simulink model "dab_bidirectional_converter_model"  (R2024a)
settings: Solver=ode23tb  StartTime=0.0  StopTime=0.5  MaxStep=1e-3  RelTol=1e-3  EnableMultiTasking=on
PreLoadFcn:
  | DualActiveBridgeConverterData
undefined symbols (not defined in the file): Ts_Power
libraries: spsMosfetLib x8, spsSeriesRLCBranchLib x7, spsVoltageMeasurementLib x5, spsCurrentMeasurementLib x3, simulink_extras x2, spsSawtoothGeneratorLib x2, spsMeanLib x2, spsDCVoltageSourceLib x2, spsLinearTransformerLib x1, slpidlib x1, spsStairGeneratorLib x1, spspowerguiLib x1
settings Model: SimulationMode=accelerator  Creator=The MathWorks, Inc.  LastModifiedBy=hamza
settings SolverCC: AlgebraicLoopSolver=TrustRegion
settings DataIOCC: LimitDataPoints=on  SaveFormat=Array  SaveOutput=off  DSMLogging=off  SaveTime=off  ReturnWorkspaceOutputs=off
settings OptimizationCC: LifeSpan=inf
settings DebuggingCC: SaveWithParameterizedLinksMsg=none  UnderspecifiedInitializationDetection=Classic  MergeDetectMultiDrivingBlocksExec=none  SolverPrmCheckMsg=warning  FcnCallInpInsideContextMsg=warning  UnconnectedInputMsg=warning  UnconnectedOutputMsg=warning  UnconnectedLineMsg=warning  StateNameClashWarn=warning  SubsystemReferenceDiagnosticForUnitTest=warning  SFUnexpectedBacktrackingDiag=warning  SFNoUnconditionalDefaultTransitionDiag=warning  SFExecutionAtInitializationDiag=none  ArithmeticOperatorsInVariantConditions=warning
settings HardwareCC: ProdBitPerPointer=32  ProdBitPerSizeT=32  ProdBitPerPtrDiffT=32  ProdLargestAtomicFloat=None  ProdIntDivRoundTo=Undefined  ProdEndianess=Unspecified  ProdWordSize=32  ProdHWDeviceType=32-bit Generic  TargetHWDeviceType=32-bit Generic
settings ModelReferenceCC: EnableRefExpFcnMdlSchedulingChecks=on  PropagateSignalLabelsOutOfModel=off
settings SFSimCC: SimUseLocalCustomCode=off  CustomCodeUndefinedFunction=UseInterfaceOnly
settings RTWCC: RTWUseLocalCustomCode=off  GPUComputeCapability=3.5  DLArmComputeVersion=19.05
settings CodeAppCC: StateflowObjectComments=on
settings GRTTargetCC: TargetFcnLib=ansi_tfl_tmw.mat  TargetLangStandard=C89/C90 (ANSI)  CombineOutputUpdateFcns=off  GRTInterface=on
settings ConfigComp: CovMetricSettings=dw  CovSaveCumulativeToWorkspaceVar=on  CovSaveSingleToWorkspaceVar=on  CovExternalEMLEnable=off  CovSFcnEnable=off

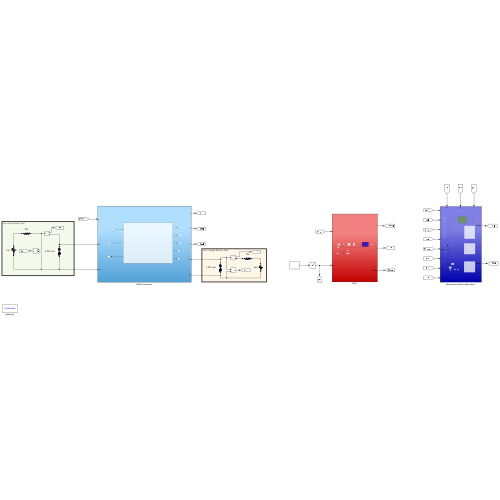
[thumbnail: Simulink's stored preview of the top-level diagram]
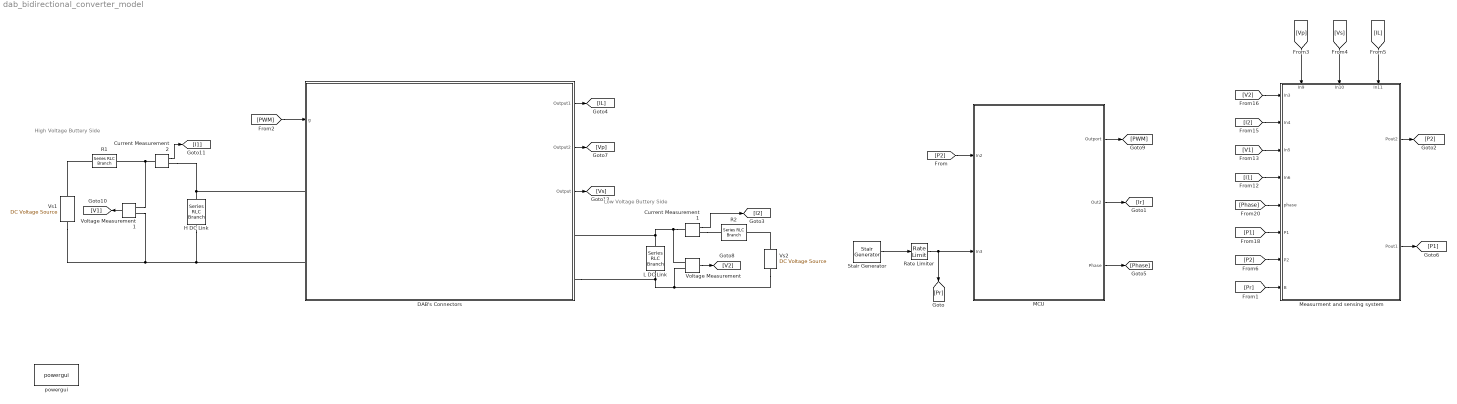
== system dab_bidirectional_converter_model ==
  note: Low Voltage Buttery Side
  note: High Voltage Buttery Side
  Current Measurement1 : spsCurrentMeasurementLib/Current Measurement  PhasorSimulation=off  OutputType=Complex  PSBequivalent=0
  Current Measurement2 : spsCurrentMeasurementLib/Current Measurement  PhasorSimulation=off  OutputType=Complex  PSBequivalent=0
  "DAB's Connectors " : Subsystem
  H DC Link : spsSeriesRLCBranchLib/Series RLC Branch  LConnTagsString=__new0  RConnTagsString=__new0  BranchType=RC  Resistance=1e-3  Inductance=1  SetiL0=off  InitialCurrent=0  Capacitance=100e-5  Setx0=off  InitialVoltage=0  Measurements=None
  L DC Link : spsSeriesRLCBranchLib/Series RLC Branch  LConnTagsString=__new0  RConnTagsString=__new0  BranchType=RC  Resistance=1e-3  Inductance=1  SetiL0=off  InitialCurrent=0  Capacitance=100e-5  Setx0=off  InitialVoltage=0  Measurements=None
  MCU : Subsystem
  Measurment and sensing system : Subsystem
      settings: PortSchema="{\"entries\":[{\"content\":{\"sides\":[{\"content\":{\"connectorIds\":[\"In1\",\"In2\",\"In3\",\"In4\",\"In5\",\"In6\",\"In7\",\"In8\"]},\"type\":\"ConnectorPlacement.EquallySpacedRectSide\",\"uuid\":\"21238e19-9896-4fd6-b727-7e2844941531\"},{\"content\":{\"connectorIds\":[\"Out1\",\"Out2\"],\"side\":\"RIGHT\"},\"type\":\"ConnectorPlacement.EquallySpacedRectSide\",\"uuid\":\"ba89ef00-1c8d-4ed8-ad10-17dc1dc7ec4f\"},{\"content\":{\"connectorIds\":[\"In9\",\"In10\",\"In11\"],\"side\":\"TOP\"},\"type\":\"ConnectorPlacement.EquallySpacedRectSide\",\"uuid\":\"e390a5d7-e81e-44f7-bbae-e4ebff839666\"}]},\"type\":\"ConnectorPlacement.EquallySpacedConnector\",\"uuid\":\"e20906e7-f3d4-4f84-9623-f1df5eb2e679\"}],\"packageUris\":[\"http://schema.mathworks.com/mf0/Connector/R2020b\"],\"version\":\"1.0\"}"
  R1 : spsSeriesRLCBranchLib/Series RLC Branch  LConnTagsString=__new0  RConnTagsString=__new0  BranchType=R  Resistance=20e-3  Inductance=1  SetiL0=off  InitialCurrent=0  Capacitance=1  Setx0=off  InitialVoltage=0  Measurements=None
  R2 : spsSeriesRLCBranchLib/Series RLC Branch  LConnTagsString=__new0  RConnTagsString=__new0  BranchType=R  Resistance=60e-3  Inductance=100e-6  SetiL0=off  InitialCurrent=0  Capacitance=1  Setx0=off  InitialVoltage=0  Measurements=None
  Rate Limiter : RateLimiter  RisingSlewLimit=50  FallingSlewLimit=-50  SampleTimeMode=inherited
  Stair Generator : spsStairGeneratorLib/Stair Generator  t=[0, 0.2]  e=[2 , -2.1]  Ts=0
  Voltage Measurement : spsVoltageMeasurementLib/Voltage Measurement  PhasorSimulation=off  OutputType=Complex  PSBequivalent=0
  Voltage Measurement1 : spsVoltageMeasurementLib/Voltage Measurement  PhasorSimulation=off  OutputType=Complex  PSBequivalent=0
  Vs1 : spsDCVoltageSourceLib/DC Voltage Source  Amplitude=400  Measurements=None
  Vs2 : spsDCVoltageSourceLib/DC Voltage Source  Amplitude=45  Measurements=None
  powergui : spspowerguiLib/powergui  Priority=1  SimulationMode=Continuous  SampleTime=Ts_Power  frequency=60  Iterations=50  frequencyindice=0  Pbase=100e6  ErrMax=1e-4  UnitsV=kV  UnitsW=MW  buscounter=0  FunctionMessages=off  echomessages=off  EnableUseOfTLC=off  CurrentSourceSwitches=on  DisableSnubberDevices=off  DisableRonSwitches=off  DisableVfSwitches=off  DisplayEquations=off  AutomaticDiscreteSolvers=off  SolverType=Tustin/Backward Euler (TBE)  Interpol=off  ExternalGateDelay=off  methode=off  Ts=10  x0status=blocks  SPID=on  SwTol=0  HookPort=off  NonlinearTolerance=1e-4  nMaxIteration=100  ContinueOnMaxIteration=off  RestoreLinks=warning  ResistiveCurrentMeasurement=off  Frange=[0:2:500]  Ylog=off  Xlog=on  ShowGrid=off  save=off  variable=ZData  structure=0  ZoomFFT=off  StartTime=0.0  cycles=1  DisplayStyle=1  fundamental=60  FreqAxis=off  MaxFrequency=1000  frequencyindicesteady=1  RmsSteady=1  display=off
  wires:
  [V2] -> Measurment and sensing system/1(In3)
  [I2] -> Measurment and sensing system/2(In4)
  [V1] -> Measurment and sensing system/3(In5)
  [I1] -> Measurment and sensing system/4(In6)
  [Phase] -> Measurment and sensing system/5(phase)
  [P1] -> Measurment and sensing system/6(P1)
  [P2] -> Measurment and sensing system/7(P2)
  Measurment and sensing system/1(Pout2) -> [P2]
  Measurment and sensing system/2(Pout1) -> [P1]
  [P2] -> MCU/1(In2)
  MCU/1(Outport) -> [PWM]
  MCU/3(Phase) -> [Phase]
  [PWM] -> "DAB's Connectors "/1(g)
  Current Measurement2/1 -> [I1]
  MCU/2(Out2) -> [Ir]
  "DAB's Connectors "/1(Output1) -> [IL]
  "DAB's Connectors "/2(Output2) -> [Vp]
  "DAB's Connectors "/3(Output) -> [Vs]
  [Vs] -> Measurment and sensing system/10(In10)
  [Vp] -> Measurment and sensing system/9(In9)
  [IL] -> Measurment and sensing system/11(In11)
  Stair Generator/1 -> Rate Limiter/1
  Rate Limiter/1 -> MCU/2(In3), [Pr]
  [Pr] -> Measurment and sensing system/8(B)
  Voltage Measurement1/1 -> [V1]
  Current Measurement1/1 -> [I2]
  Voltage Measurement/1 -> [V2]
  connections:
  Current Measurement2/RConn1 -- "DAB's Connectors "/LConn1 -- H DC Link/RConn1
  H DC Link/LConn1 -- Voltage Measurement1/LConn2 -- Vs1/LConn1 -- "DAB's Connectors "/LConn2
  R1/LConn1 -- Voltage Measurement1/LConn1 -- Current Measurement2/LConn1
  R1/RConn1 -- Vs1/RConn1
  Current Measurement1/LConn1 -- L DC Link/RConn1 -- "DAB's Connectors "/RConn1 -- Voltage Measurement/LConn1
  Voltage Measurement/LConn2 -- "DAB's Connectors "/RConn2 -- L DC Link/LConn1 -- Vs2/LConn1
  Vs2/RConn1 -- R2/LConn1
  Current Measurement1/RConn1 -- R2/RConn1

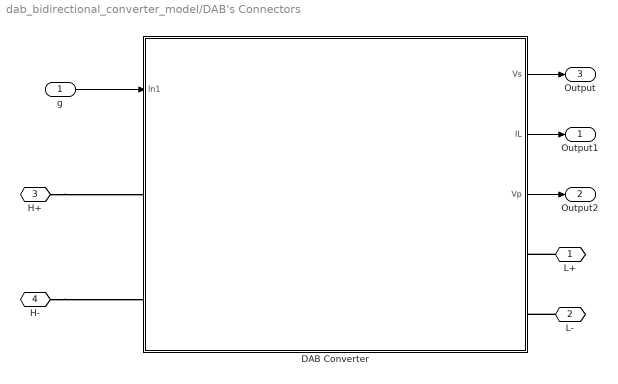
== system dab_bidirectional_converter_model/DAB's Connectors  ==
  g : Inport
  DAB Converter : Subsystem
  L+ : PMIOPort  Side=Right
  L- : PMIOPort  Port=2  Side=Right
  H+ : PMIOPort  Port=3  Side=Left
  H- : PMIOPort  Port=4  Side=Left
  Output1 : Outport
  Output2 : Outport  Port=2
  Output : Outport  Port=3
  wires:
  g/1 -> DAB Converter/1(In1)
  DAB Converter/1(Vs) -> Output/1
  DAB Converter/2(IL) -> Output1/1
  DAB Converter/3(Vp) -> Output2/1
  connections:
  H+/RConn1 -- DAB Converter/LConn1
  H-/RConn1 -- DAB Converter/LConn2
  L-/RConn1 -- DAB Converter/RConn2
  L+/RConn1 -- DAB Converter/RConn1

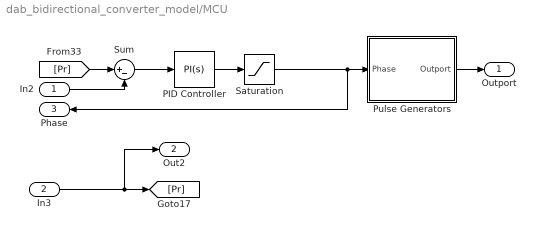
== system dab_bidirectional_converter_model/MCU ==
  In2 : Inport
  In3 : Inport  Port=2
  PID Controller : slpidlib/PID Controller  Controller=PI  Form=Parallel  TimeDomain=Continuous-time  UseExternalTs=off  SampleTime=-1  IntegratorMethod=Forward Euler  FilterMethod=Forward Euler  ControllerParametersSource=internal  P=0.1  I=600  UseKiTs=off  D=0  UseExternalDerivativeSource=off  N=100  UseFilter=on  TunerSelectOption=Transfer Function Based (PID Tuner App)  InitialConditionSource=internal  InitialConditionForIntegrator=0  InitialConditionForFilter=0  DifferentiatorICPrevScaledInput=0  ExternalReset=none  TrackingMode=off  Kt=1  LimitOutput=off  SatLimitsSource=internal  UpperSaturationLimit=inf  LowerSaturationLimit=-inf  LinearizeAsGain=on  AntiWindupMode=none  Kb=1  LimitIntegrator=off  UpperIntegratorSaturationLimit=inf  LowerIntegratorSaturationLimit=-inf  POutMin=[]  POutMax=[]  IOutMin=[]  IOutMax=[]  DOutMin=[]  DOutMax=[]  NOutMin=[]  NOutMax=[]  SumOutMin=[]  SumOutMax=[]  SaturationOutMin=[]  SaturationOutMax=[]  PParamMin=[]  PParamMax=[]  IParamMin=[]  IParamMax=[]  DParamMin=[]  DParamMax=[]  NParamMin=[]  NParamMax=[]  KbParamMin=[]  KbParamMax=[]  KtParamMin=[]  KtParamMax=[]  KbOutMin=[]  KbOutMax=[]  KtOutMin=[]  KtOutMax=[]  IntegratorOutMin=[]  IntegratorOutMax=[]  FilterOutMin=[]  FilterOutMax=[]  SumI1OutMin=[]  SumI1OutMax=[]  SumI2OutMin=[]  SumI2OutMax=[]  SumI3OutMin=[]  SumI3OutMax=[]  SumI4OutMin=[]  SumI4OutMax=[]  SumDOutMin=[]  SumDOutMax=[]  DifferentiatorOutMin=[]  DifferentiatorOutMax=[]  FilterDiffOutCoefMin=[]  FilterDiffOutCoefMax=[]  ReciprocalOutMin=[]  ReciprocalOutMax=[]  SumDenOutMin=[]  SumDenOutMax=[]  SumNumOutMin=[]  SumNumOutMax=[]  DivideOutMin=[]  DivideOutMax=[]  UdiffTsProdOutMin=[]  UdiffTsProdOutMax=[]  NTsProdOutMin=[]  NTsProdOutMax=[]  UintegralTsProdOutMin=[]  UintegralTsProdOutMax=[]  UngainTsProdOutMin=[]  UngainTsProdOutMax=[]  ClampingZeroOutDataTypeStr=Inherit: Inherit via back propagation  ClampingZeroOutMin=[]  ClampingZeroOutMax=[]  FilterDenConstantOutDataTypeStr=Inherit: Inherit via back propagation  FilterDenConstantOutMin=[]  FilterDenConstantOutMax=[]  PCopyOutDataTypeStr=Inherit: Inherit via back propagation  PCopyOutMin=[]  PCopyOutMax=[]  NCopyOutDataTypeStr=Inherit: Inherit via back propagation  NCopyOutMin=[]  NCopyOutMax=[]  IntegratorContinuousStateAttributes=''  IntegratorStateMustResolveToSignalObject=off  IntegratorRTWStateStorageClass=Auto  FilterContinuousStateAttributes=''  FilterStateMustResolveToSignalObject=off  FilterRTWStateStorageClass=Auto  ParallelPVariant=InternalParameters  IdealPVariant=Disabled  IVariant=InternalParameters  DVariant=Disabled  IntegratorVariant=Continuous  SatVariant=Disabled  AWVariant=Passthrough  PCopyVariant=Disabled  TRVariant=Disabled  FdbkBlocksVariant=Forward  IdealPFdbkVariant=Disabled  SatFdbkVariant=Disabled  DerivativeFilterVariant=Disabled  NVariant=Disabled  NCopyVariant=Disabled_SignalSpec  FilterICVariant=Disabled  IntegratorICVariant=InternalICs  ExternalResetVariant=Disabled  TRSumVariant=Passthrough  SumFdbkVariant=Disabled  SumVariant=Sum_PI  TsampFilterVariant=InternalTs  TsampNgainVariant=Passthrough  TsampIntegralVariant=Disabled_SignalSpec  ExternalSaturationOutDataTypeStr=Inherit: Same as second input  DerivativeSourceVariant=Disabled
  Pulse Generators : Subsystem
  Saturation : Saturate  UpperLimit=35  LowerLimit=-35
  Sum : Sum  Inputs=|+-
  Outport : Outport
  Out2 : Outport  Port=2
  Phase : Outport  Port=3
  wires:
  In3/1 -> Out2/1, [Pr]
  Pulse Generators/1(Outport) -> Outport/1
  [Pr] -> Sum/1
  In2/1 -> Sum/2
  PID Controller/1 -> Saturation/1
  Sum/1 -> PID Controller/1
  Saturation/1 -> Phase/1, Pulse Generators/1(Phase)

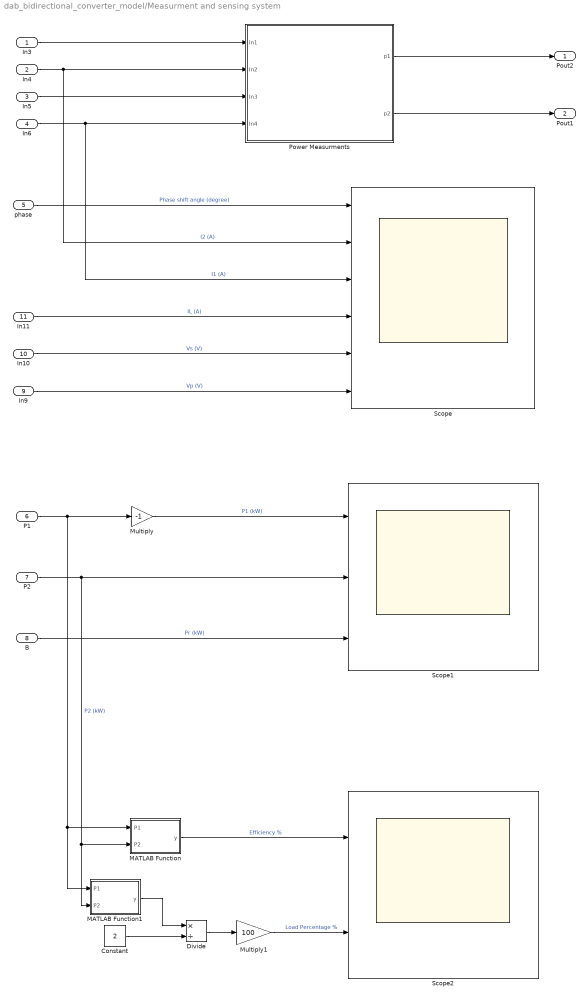
== system dab_bidirectional_converter_model/Measurment and sensing system ==
  In3 : Inport
  In4 : Inport  Port=2
  In5 : Inport  Port=3
  In6 : Inport  Port=4
  phase : Inport  Port=5
  P1 : Inport  Port=6
  P2 : Inport  Port=7
  B : Inport  Port=8
  In9 : Inport  Port=9
  In10 : Inport  Port=10
  In11 : Inport  Port=11
  Constant : Constant  Value=2
  Divide : Product  Inputs=*/
  MATLAB Function : MATLAB Function  TreatAsAtomicUnit=on
  MATLAB Function1 : MATLAB Function  TreatAsAtomicUnit=on
  Multiply : Gain  Gain=-1
  Multiply1 : Gain  Gain=100
  Power Measurments : Subsystem
  Scope : Scope  NumInputPorts=6
  Scope1 : Scope  NumInputPorts=3
  Scope2 : Scope  NumInputPorts=2
  Pout2 : Outport
  Pout1 : Outport  Port=2
  wires:
  P2/1 -> MATLAB Function1/2(P2), MATLAB Function/2(P2), Scope1/2  "P2 (kW)"
  In4/1 -> Scope/2, Power Measurments/2(In2)  "I2 (A)"
  phase/1 -> Scope/1  "Phase shift angle (degree)"
  P1/1 -> MATLAB Function1/1(P1), MATLAB Function/1(P1), Multiply/1
  In3/1 -> Power Measurments/1(In1)
  In5/1 -> Power Measurments/3(In3)
  In6/1 -> Scope/3, Power Measurments/4(In4)  "I1 (A)"
  Power Measurments/1(p1) -> Pout2/1
  Power Measurments/2(p2) -> Pout1/1
  B/1 -> Scope1/3  "Pr (kW)"
  Multiply/1 -> Scope1/1  "P1 (kW)"
  In9/1 -> Scope/6  "Vp (V)"
  In10/1 -> Scope/5  "Vs (V)"
  In11/1 -> Scope/4  "IL (A)"
  Constant/1 -> Divide/2
  Divide/1 -> Multiply1/1
  Multiply1/1 -> Scope2/2  "Load Percentage %"
  MATLAB Function/1(y) -> Scope2/1  "Efficiency %"
  MATLAB Function1/1(y) -> Divide/1

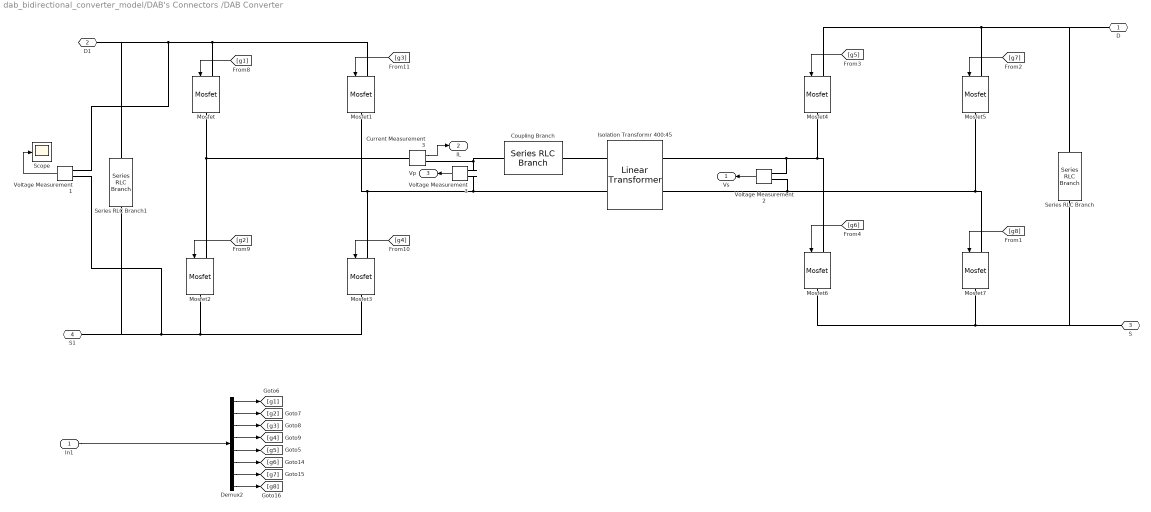
== system dab_bidirectional_converter_model/DAB's Connectors /DAB Converter ==
  In1 : Inport
  Coupling Branch : spsSeriesRLCBranchLib/Series RLC Branch  LConnTagsString=__new0  RConnTagsString=__new0  BranchType=RL  Resistance=4.5e-3  Inductance=100e-6  SetiL0=off  InitialCurrent=0  Capacitance=1e-6  Setx0=off  InitialVoltage=0  Measurements=None
  Current Measurement3 : spsCurrentMeasurementLib/Current Measurement  PhasorSimulation=off  OutputType=Complex  PSBequivalent=0
  Demux2 : Demux  Outputs=8
  Isolation Transformr 400:45 : spsLinearTransformerLib/Linear Transformer  UNITS=SI  NominalPower="[ 2e3,  50e3]"  winding1=[400, 10e-3, 15e-6]  winding2=[45, 1e-6, 0]  ThreeWindings=off  winding3=[3.15e+05 0.7938 0.084225]  RmLm="[ 10e3,  16e-3]"  Measurements=None  DataType=on
  Mosfet{,1..7} (8 alike) : spsMosfetLib/Mosfet  Ron=11e-3  Lon=0  Rd=10e-3  Vfd=0.9  IC=0  Rs=1e6  Cs=inf  Measurements=off
  Scope : Scope
  Series RLC Branch : spsSeriesRLCBranchLib/Series RLC Branch  LConnTagsString=__new0  RConnTagsString=__new0  BranchType=C  Resistance=1  Inductance=1e-3  SetiL0=off  InitialCurrent=0  Capacitance=1e-3  Setx0=off  InitialVoltage=0  Measurements=None
  Series RLC Branch1 : spsSeriesRLCBranchLib/Series RLC Branch  LConnTagsString=__new0  RConnTagsString=__new0  BranchType=C  Resistance=1  Inductance=1e-3  SetiL0=off  InitialCurrent=0  Capacitance=1e-3  Setx0=off  InitialVoltage=0  Measurements=None
  Voltage Measurement1 : spsVoltageMeasurementLib/Voltage Measurement  PhasorSimulation=off  OutputType=Complex  PSBequivalent=0
  Voltage Measurement2 : spsVoltageMeasurementLib/Voltage Measurement  PhasorSimulation=off  OutputType=Complex  PSBequivalent=0
  Voltage Measurement3 : spsVoltageMeasurementLib/Voltage Measurement  PhasorSimulation=off  OutputType=Complex  PSBequivalent=0
  D : PMIOPort  Side=Right
  D1 : PMIOPort  Port=2  Side=Left
  S : PMIOPort  Port=3  Side=Right
  S1 : PMIOPort  Port=4  Side=Left
  Vs : Outport
  IL : Outport  Port=2
  Vp : Outport  Port=3
  wires:
  In1/1 -> Demux2/1
  Demux2/3 -> [g3]
  Voltage Measurement3/1 -> Vp/1
  Demux2/2 -> [g2]
  Current Measurement3/1 -> IL/1
  [g7] -> Mosfet5/1
  [g8] -> Mosfet7/1
  [g5] -> Mosfet4/1
  Demux2/6 -> [g6]
  [g2] -> Mosfet2/1
  Demux2/8 -> [g8]
  Demux2/4 -> [g4]
  Demux2/7 -> [g7]
  Demux2/1 -> [g1]
  Voltage Measurement2/1 -> Vs/1
  [g6] -> Mosfet6/1
  Demux2/5 -> [g5]
  [g3] -> Mosfet1/1
  [g4] -> Mosfet3/1
  [g1] -> Mosfet/1
  Voltage Measurement1/1 -> Scope/1
  connections:
  Isolation Transformr 400:45/LConn1 -- Coupling Branch/RConn1
  Isolation Transformr 400:45/RConn2 -- Mosfet7/LConn1 -- Mosfet5/RConn1 -- Voltage Measurement2/LConn2
  Mosfet4/LConn1 -- Series RLC Branch/LConn1 -- D/RConn1 -- Mosfet5/LConn1
  Mosfet/LConn1 -- Voltage Measurement1/LConn1 -- D1/RConn1 -- Series RLC Branch1/LConn1 -- Mosfet1/LConn1
  Isolation Transformr 400:45/RConn1 -- Voltage Measurement2/LConn1 -- Mosfet6/LConn1 -- Mosfet4/RConn1
  Voltage Measurement3/LConn2 -- Isolation Transformr 400:45/LConn2 -- Mosfet3/LConn1 -- Mosfet1/RConn1
  Current Measurement3/RConn1 -- Coupling Branch/LConn1 -- Voltage Measurement3/LConn1
  Mosfet6/RConn1 -- Series RLC Branch/RConn1 -- S/RConn1 -- Mosfet7/RConn1
  Mosfet2/RConn1 -- Voltage Measurement1/LConn2 -- Series RLC Branch1/RConn1 -- S1/RConn1 -- Mosfet3/RConn1
  Current Measurement3/LConn1 -- Mosfet/RConn1 -- Mosfet2/LConn1

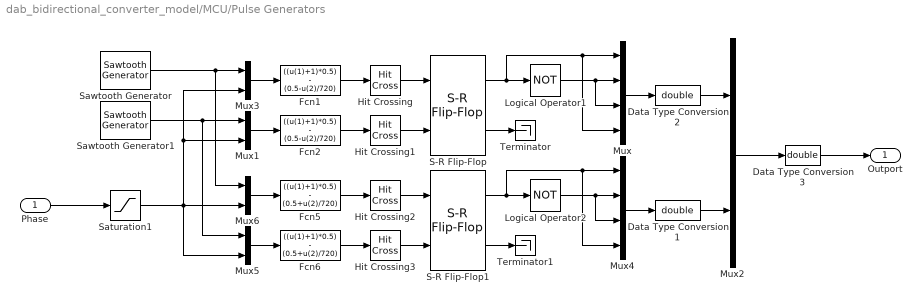
== system dab_bidirectional_converter_model/MCU/Pulse Generators ==
  Phase : Inport
  Data Type Conversion1 : DataTypeConversion  OutDataTypeStr=double  SaturateOnIntegerOverflow=off  RndMeth=Floor
  Data Type Conversion2 : DataTypeConversion  OutDataTypeStr=double  SaturateOnIntegerOverflow=off  RndMeth=Floor
  Data Type Conversion3 : DataTypeConversion  OutDataTypeStr=double  SaturateOnIntegerOverflow=off  RndMeth=Floor
  Fcn1 : Fcn  Expr=((u(1)+1)*0.5) - (0.5-u(2)/720)
  Fcn2 : Fcn  Expr=((u(1)+1)*0.5) - (0.5-u(2)/720)
  Fcn5 : Fcn  Expr=((u(1)+1)*0.5) - (0.5+u(2)/720)
  Fcn6 : Fcn  Expr=((u(1)+1)*0.5) - (0.5+u(2)/720)
  Hit Crossing{,1..3} (4 alike) : HitCross  HitCrossingDirection=rising
  Logical Operator1 : Logic  Operator=NOT  AllPortsSameDT=off  OutDataTypeStr=boolean
  Logical Operator2 : Logic  Operator=NOT  AllPortsSameDT=off  OutDataTypeStr=boolean
  Mux : Mux
  Mux{1,3,5..6} (4 alike) : Mux  Inputs=2
  Mux2 : Mux  Inputs=[4,4]
  Mux4 : Mux
  S-R Flip-Flop : simulink_extras/Flip Flops/S-R Flip-Flop  initial_condition=0
  S-R Flip-Flop1 : simulink_extras/Flip Flops/S-R Flip-Flop  initial_condition=0
  Saturation1 : Saturate  UpperLimit=180  LowerLimit=-180
  Sawtooth Generator : spsSawtoothGeneratorLib/Sawtooth Generator  Freq=50e3  Phase=0  Ts=0
  Sawtooth Generator1 : spsSawtoothGeneratorLib/Sawtooth Generator  Freq=50e3  Phase=180  Ts=0
  Terminator : Terminator
  Terminator1 : Terminator
  Outport : Outport
  wires:
  Logical Operator1/1 -> Mux/2, Mux/3
  Sawtooth Generator/1 -> Mux6/1, Mux3/1
  Fcn1/1 -> Hit Crossing/1
  Fcn2/1 -> Hit Crossing1/1
  Hit Crossing/1 -> S-R Flip-Flop/1
  Hit Crossing1/1 -> S-R Flip-Flop/2
  S-R Flip-Flop/1 -> Mux/4, Mux/1, Logical Operator1/1
  S-R Flip-Flop/2 -> Terminator/1
  Mux/1 -> Data Type Conversion2/1
  Data Type Conversion2/1 -> Mux2/1
  Data Type Conversion1/1 -> Mux2/2
  Mux3/1 -> Fcn1/1
  Mux1/1 -> Fcn2/1
  Saturation1/1 -> Mux6/2, Mux5/2, Mux1/2, Mux3/2
  Mux5/1 -> Fcn6/1
  Mux6/1 -> Fcn5/1
  Mux4/1 -> Data Type Conversion1/1
  S-R Flip-Flop1/2 -> Terminator1/1
  S-R Flip-Flop1/1 -> Logical Operator2/1, Mux4/1, Mux4/4
  Hit Crossing3/1 -> S-R Flip-Flop1/2
  Hit Crossing2/1 -> S-R Flip-Flop1/1
  Fcn6/1 -> Hit Crossing3/1
  Fcn5/1 -> Hit Crossing2/1
  Logical Operator2/1 -> Mux4/3, Mux4/2
  Sawtooth Generator1/1 -> Mux5/1, Mux1/1
  Mux2/1 -> Data Type Conversion3/1
  Phase/1 -> Saturation1/1
  Data Type Conversion3/1 -> Outport/1

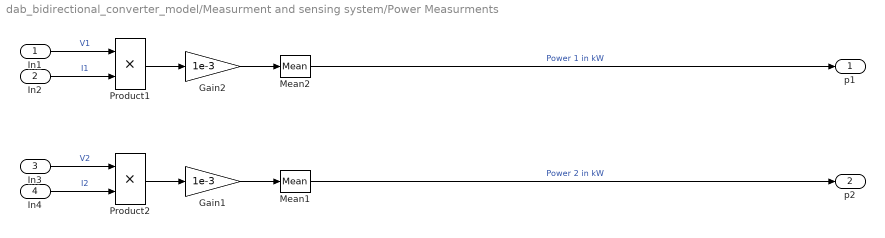
== system dab_bidirectional_converter_model/Measurment and sensing system/Power Measurments ==
  In1 : Inport
  In2 : Inport  Port=2
  In3 : Inport  Port=3
  In4 : Inport  Port=4
  Gain1 : Gain  Gain=1e-3
  Gain2 : Gain  Gain=1e-3
  Mean1 : spsMeanLib/Mean  Freq=50e3  Vinit=0  Ts=0
  Mean2 : spsMeanLib/Mean  Freq=50e3  Vinit=0  Ts=0
  Product1 : Product
  Product2 : Product
  p1 : Outport
  p2 : Outport  Port=2
  wires:
  In1/1 -> Product1/1  "V1"
  Product1/1 -> Gain2/1
  Gain2/1 -> Mean2/1
  In3/1 -> Product2/1  "V2"
  Mean1/1 -> p2/1  "Power 2 in kW"
  In4/1 -> Product2/2  "I2"
  Product2/1 -> Gain1/1
  Gain1/1 -> Mean1/1
  In2/1 -> Product1/2  "I1"
  Mean2/1 -> p1/1  "Power 1 in kW"

== matlab function dab_bidirectional_converter_model/Measurment and sensing system/MATLAB Function ==
  data: P1 input; y output; P2 input
function y = fcn(P1, P2)
  
    if P1 == 0 && P2 == 0 %% to avoid undifiened statues
        y = 0; 
        return;
    end

    if P1 == 0
        y = 0;
        return;
    elseif P2 == 0
        y = 0; 
        return;
    end

    x = abs(P2 / P1);

    if x > 1
        y = (1/x) * 100; 
    else
        y = (x) * 100; 
    end
end

== matlab function dab_bidirectional_converter_model/Measurment and sensing system/MATLAB Function1 ==
  data: P1 input; y output; P2 input
function y = fcn(P1,P2)

if abs(P1)>= abs(P2)
y = abs(P2);

else 
y=abs(P1);

end
